simulink model "SimCurtoCircuitoMeioLinhaSemCompensacao"  (R2021b)
settings: Solver=ode45  StartTime=0.0  StopTime=0.1  RelTol=1e-3  EnableMultiTasking=on
values from neighbouring files (symbols this model uses):
  le = 1e-10    [RotinaCurtoCircuitoCompacto.m]    (also in RotinaCurtoCircuitoCompleta.m; RotinaCurtoCircuitoT2F_Trifasico.m)
  lm = (imag(Zm)/(2*pi*f))*d    [RotinaCurtoCircuitoCompacto.m]    (also in RotinaCurtoCircuitoCompleta.m; RotinaCurtoCircuitoT2F_Trifasico.m)
  lp = (imag(Zp)/(2*pi*f))*d    [RotinaCurtoCircuitoCompacto.m]    (also in RotinaCurtoCircuitoCompleta.m; RotinaCurtoCircuitoT2F_Trifasico.m)
  m1 = n    [RotinaCurtoCircuitoCompacto.m]    (also in RotinaCurtoCircuitoCompleta.m; RotinaCurtoCircuitoT2F_Trifasico.m)
  m2 = 1 - m1    [RotinaCurtoCircuitoCompacto.m]    (also in RotinaCurtoCircuitoCompleta.m; RotinaCurtoCircuitoT2F_Trifasico.m)
  NRE = 1e-12    [RotinaCurtoCircuitoCompacto.m]    (also in RotinaCurtoCircuitoCompleta.m; RotinaCurtoCircuitoT2F_Trifasico.m)
  Raf = 1e6    (= 1000000)    [RotinaCurtoCircuitoCompacto.m]    (also in RotinaCurtoCircuitoCompleta.m; RotinaCurtoCircuitoT2F_Trifasico.m = 100000)
  Rbf = 1e6    (= 1000000)    [RotinaCurtoCircuitoCompacto.m]    (also in RotinaCurtoCircuitoCompleta.m; RotinaCurtoCircuitoT2F_Trifasico.m = 1e-05)
  Rcf = 1e6    (= 1000000)    [RotinaCurtoCircuitoCompacto.m]    (also in RotinaCurtoCircuitoCompleta.m; RotinaCurtoCircuitoT2F_Trifasico.m = 1e-05)
  rm = real(Zm)*d    [RotinaCurtoCircuitoCompacto.m]    (also in RotinaCurtoCircuitoCompleta.m; RotinaCurtoCircuitoT2F_Trifasico.m)
  rp = real(Zp)*d    [RotinaCurtoCircuitoCompacto.m]    (also in RotinaCurtoCircuitoCompleta.m; RotinaCurtoCircuitoT2F_Trifasico.m)
  rtc = 10    [RotinaCurtoCircuitoCompacto.m]    (also in RotinaCurtoCircuitoCompleta.m; RotinaCurtoCircuitoT2F_Trifasico.m)
  rti = 10    [RotinaCurtoCircuitoCompacto.m]    (also in RotinaCurtoCircuitoCompleta.m; RotinaCurtoCircuitoT2F_Trifasico.m)
undefined symbols (not defined in the file or in its folder): D11, Delta
libraries: spsSeriesRLCBranchLib x6, spsThreePhaseVIMeasurementLib x2, spsThreePhaseTransformerTwoWindingsLib x2, spsVoltageMeasurementLib x2, spsMutualInductanceLib x2, spsThreePhaseSourceLib x1, spspowerguiLib x1
settings Model: Creator=laris  LastModifiedBy=LeonardoFelipe
settings SolverCC: AlgebraicLoopSolver=TrustRegion
settings DataIOCC: LimitDataPoints=on  SaveFormat=Array  ReturnWorkspaceOutputs=off
settings OptimizationCC: LifeSpan=inf
settings DebuggingCC: SFUnexpectedBacktrackingDiag=warning  SFNoUnconditionalDefaultTransitionDiag=warning  SFExecutionAtInitializationDiag=none  SFMachineParentedDataDiag=warning  ArithmeticOperatorsInVariantConditions=warning
settings HardwareCC: ProdBitPerPointer=32  ProdBitPerSizeT=32  ProdBitPerPtrDiffT=32  ProdLargestAtomicFloat=None  ProdIntDivRoundTo=Undefined  ProdEndianess=Unspecified  ProdWordSize=32  ProdHWDeviceType=32-bit Generic
settings ModelReferenceCC: PropagateSignalLabelsOutOfModel=off
settings SFSimCC: SimUseLocalCustomCode=off  CustomCodeUndefinedFunction=UseInterfaceOnly
settings RTWCC: RTWUseLocalCustomCode=off
settings CodeAppCC: StateflowObjectComments=on
settings GRTTargetCC: TargetLangStandard=C89/C90 (ANSI)
settings ConfigComp: CovMetricSettings=dw  CovSaveCumulativeToWorkspaceVar=on  CovSaveSingleToWorkspaceVar=on  CovExternalEMLEnable=off
settings SimscapeCC: SimscapeNormalizeSystem=off

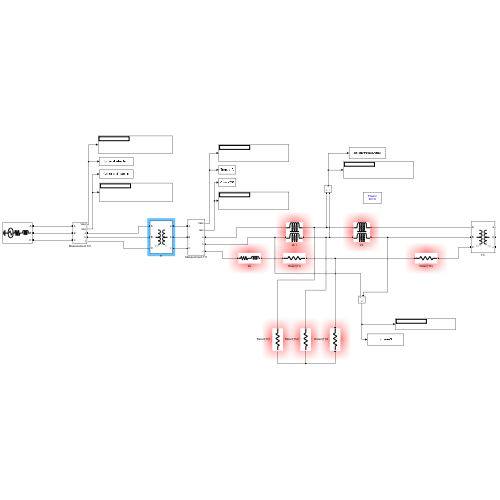
[thumbnail: Simulink's stored preview of the top-level diagram]
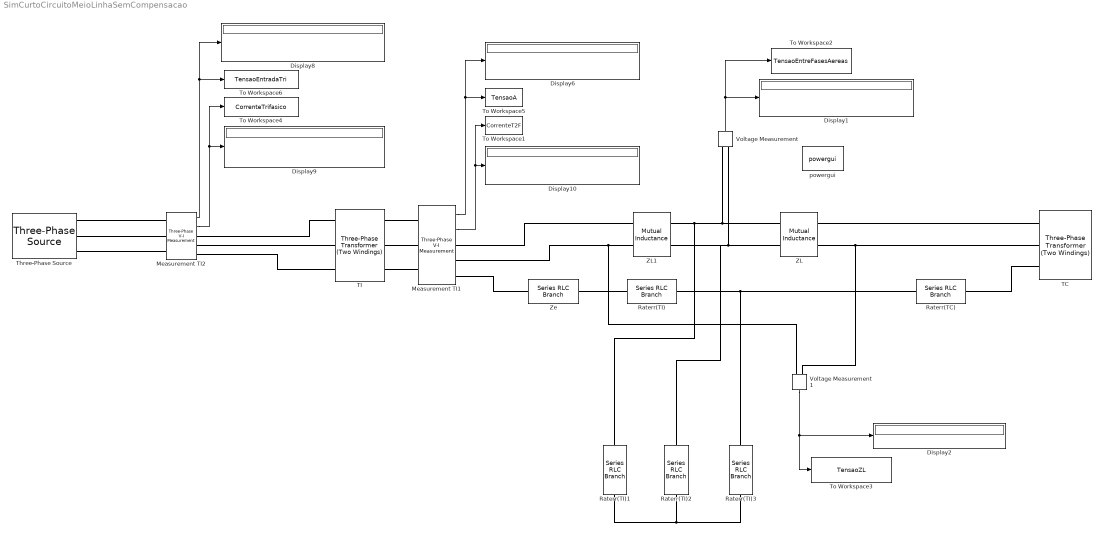
== system SimCurtoCircuitoMeioLinhaSemCompensacao ==
  Display{1..2,6,8..10} (6 alike) : Display
  Measurement TI1 : spsThreePhaseVIMeasurementLib/Three-Phase V-I Measurement  VoltageMeasurement=phase-to-phase  SetLabelV=off  LabelV=Vabc  Vpu=off  VpuLL=off  CurrentMeasurement=yes  SetLabelI=off  LabelI=Iabc  Ipu=off  Pbase=100e6  Vbase=500e3  OutputType=Complex  PhasorSimulation=on  PSBequivalent=0
  Measurement TI2 : spsThreePhaseVIMeasurementLib/Three-Phase V-I Measurement  VoltageMeasurement=phase-to-ground  SetLabelV=off  LabelV=Vabc  Vpu=off  VpuLL=off  CurrentMeasurement=yes  SetLabelI=off  LabelI=Iabc  Ipu=off  Pbase=100e6  Vbase=500e3  OutputType=Complex  PhasorSimulation=on  PSBequivalent=0
  Raterr(TC) : spsSeriesRLCBranchLib/Series RLC Branch  LConnTagsString=__new0  RConnTagsString=__new0  BranchType=R  Resistance=rtc  Inductance=0  SetiL0=off  InitialCurrent=0  Capacitance=1e-6  Setx0=off  InitialVoltage=0  Measurements=None
  Raterr(TI) : spsSeriesRLCBranchLib/Series RLC Branch  LConnTagsString=__new0  RConnTagsString=__new0  BranchType=R  Resistance=rti  Inductance=0  SetiL0=off  InitialCurrent=0  Capacitance=1e-6  Setx0=off  InitialVoltage=0  Measurements=None
  Raterr(TI)1 : spsSeriesRLCBranchLib/Series RLC Branch  LConnTagsString=__new0  RConnTagsString=__new0  BranchType=R  Resistance=Raf  Inductance=0  SetiL0=off  InitialCurrent=0  Capacitance=1e-6  Setx0=off  InitialVoltage=0  Measurements=None
  Raterr(TI)2 : spsSeriesRLCBranchLib/Series RLC Branch  LConnTagsString=__new0  RConnTagsString=__new0  BranchType=R  Resistance=Rbf  Inductance=0  SetiL0=off  InitialCurrent=0  Capacitance=1e-6  Setx0=off  InitialVoltage=0  Measurements=None
  Raterr(TI)3 : spsSeriesRLCBranchLib/Series RLC Branch  LConnTagsString=__new0  RConnTagsString=__new0  BranchType=R  Resistance=Rcf  Inductance=0  SetiL0=off  InitialCurrent=0  Capacitance=1e-6  Setx0=off  InitialVoltage=0  Measurements=None
  TC : spsThreePhaseTransformerTwoWindingsLib/Three-Phase Transformer (Two Windings)  Winding1Connection=Delta (D11)  Winding2Connection=Yg  CoreType=Three single-phase transformers  SetSaturation=off  Hysteresis=off  DataFile='hysteresis'  SetInitialFlux=off  Measurements=None  UNITS=pu  NominalPower=[120e3 , 60]  Winding1=[13800 0.0048118 0.018511]  Winding2=[380 0.0048119 0.018511]  Rm=5.801193266567229e+02*1000  Lm=8.409977380031759e+02*1000  L0=0.50001  Saturation=[0 0;0.0012545 0.01913;0.52272 0.024231]  InitialFluxes=[0.66025 -0.66025 0.57767]  BreakLoop=off  DiscreteSolver=Trapezoidal iterative  DataType=off  TransfoNumber=1
  TI : spsThreePhaseTransformerTwoWindingsLib/Three-Phase Transformer (Two Windings)  Winding1Connection=Delta (D11)  Winding2Connection=Y  CoreType=Three single-phase transformers  SetSaturation=off  Hysteresis=off  DataFile='hysteresis'  SetInitialFlux=off  Measurements=None  UNITS=pu  NominalPower=[300e3 , 60 ]  Winding1=[13800 0.0048119 0.018511]  Winding2=[13800 0.0048119 0.018511]  Rm=1.730769230769231e+03*1000  Lm=40.010686750359440*1000  L0=6.3145  Saturation=[0 0;0.0012545 0.01913;0.52272 0.024231]  InitialFluxes=[34.179 -34.179 29.906]  BreakLoop=off  DiscreteSolver=Trapezoidal iterative  DataType=off  TransfoNumber=1
  Three-Phase Source : spsThreePhaseSourceLib/Three-Phase Source  InternalConnection=Yg  VoltagePhases=off  Voltage=13.8e3  PhaseAngle=0  Voltage_phases=[25e3 25e3 25e3]/sqrt(3)  PhaseAngles_phases=[0 -120 +120]  Frequency=60  NonIdealSource=on  SpecifyImpedance=on  Resistance=0.8929  Inductance=16.58e-3  ShortCircuitLevel=120e6  BaseVoltage=13.8e3  XRratio=7  BusType=swing  Pref=10e3  Qref=0  Prefabc=[10e3, 10e3, 10e3]  Qrefabc=[0, 0, 0]  Qmin=-inf  Qmax=inf
  To Workspace1 : ToWorkspace  VariableName=CorrenteT2F  SampleTime=-1
      settings: MaxDataPoints=1
  To Workspace2 : ToWorkspace  VariableName=TensaoEntreFasesAereas  SampleTime=-1
      settings: MaxDataPoints=1
  To Workspace3 : ToWorkspace  VariableName=TensaoZL  SampleTime=-1
      settings: MaxDataPoints=1
  To Workspace4 : ToWorkspace  VariableName=CorrenteTrifasico  SampleTime=-1
      settings: MaxDataPoints=1
  To Workspace5 : ToWorkspace  VariableName=TensaoA  SampleTime=-1
      settings: MaxDataPoints=1
  To Workspace6 : ToWorkspace  VariableName=TensaoEntradaTri  SampleTime=-1
      settings: MaxDataPoints=1
  Voltage Measurement : spsVoltageMeasurementLib/Voltage Measurement  PhasorSimulation=on  OutputType=Complex  PSBequivalent=0
  Voltage Measurement1 : spsVoltageMeasurementLib/Voltage Measurement  PhasorSimulation=on  OutputType=Complex  PSBequivalent=0
  ZL : spsMutualInductanceLib/Mutual Inductance  LConnTagsString=a|b  RConnTagsString=A|B  TypeOfMutual=Generalized mutual inductance  NumberOfWindings=2  SelfImpedance1=[1.1 1.1e-03]  SelfImpedance2=[ 1.1 1.1e-03]  ThreeWindings=on  SelfImpedance3=[ 1.1 1.1e-03]  MutualImpedance=[1.0 1.0e-03]  InductanceMatrix=[lp lm ; lm lp] * m2  ResistanceMatrix=[rp rm ; rm rp] * m2  Measurements=None
      settings: SourceProductBaseCode=PS
  ZL1 : spsMutualInductanceLib/Mutual Inductance  LConnTagsString=a|b  RConnTagsString=A|B  TypeOfMutual=Generalized mutual inductance  NumberOfWindings=2  SelfImpedance1=[1.1 1.1e-03]  SelfImpedance2=[ 1.1 1.1e-03]  ThreeWindings=on  SelfImpedance3=[ 1.1 1.1e-03]  MutualImpedance=[1.0 1.0e-03]  InductanceMatrix=[lp lm ; lm lp] * m1  ResistanceMatrix=[rp rm ; rm rp] * m1  Measurements=None
      settings: SourceProductBaseCode=PS
  Ze : spsSeriesRLCBranchLib/Series RLC Branch  LConnTagsString=__new0  RConnTagsString=__new0  BranchType=RL  Resistance=NRE  Inductance=le  SetiL0=off  InitialCurrent=0  Capacitance=le  Setx0=off  InitialVoltage=0  Measurements=None
  powergui : spspowerguiLib/powergui  Priority=1  SimulationMode=Phasor  SampleTime=50e-6  frequency=60  Iterations=50  frequencyindice=60  Pbase=100e6  ErrMax=1e-4  UnitsV=kV  UnitsW=MW  buscounter=0  FunctionMessages=off  echomessages=off  EnableUseOfTLC=off  CurrentSourceSwitches=off  DisableSnubberDevices=off  DisableRonSwitches=off  DisableVfSwitches=off  DisplayEquations=off  AutomaticDiscreteSolvers=off  SolverType=Tustin/Backward Euler (TBE)  Interpol=off  ExternalGateDelay=off  methode=off  Ts=100  x0status=blocks  SPID=on  SwTol=0  HookPort=off  NonlinearTolerance=1e-4  nMaxIteration=100  ContinueOnMaxIteration=off  RestoreLinks=warning  ResistiveCurrentMeasurement=off  Frange=[0:2:500]  Ylog=off  Xlog=on  ShowGrid=off  save=off  variable=ZData  structure=0  ZoomFFT=off  StartTime=0.0  cycles=1  DisplayStyle=1  fundamental=60  FreqAxis=off  MaxFrequency=1000  frequencyindicesteady=1  RmsSteady=1  display=off
  wires:
  Measurement TI1/1 -> To Workspace5/1, Display6/1
  Measurement TI2/1 -> Display8/1, To Workspace6/1
  Measurement TI2/2 -> To Workspace4/1, Display9/1
  Measurement TI1/2 -> To Workspace1/1, Display10/1
  Voltage Measurement/1 -> To Workspace2/1, Display1/1
  Voltage Measurement1/1 -> To Workspace3/1, Display2/1
  connections:
  ZL/RConn1 -- TC/LConn1
  ZL/RConn2 -- Voltage Measurement1/LConn2 -- TC/LConn2
  Raterr(TC)/RConn1 -- TC/LConn3
  TI/RConn1 -- Measurement TI1/LConn1
  Voltage Measurement/LConn1 -- ZL1/RConn1 -- Raterr(TI)1/LConn1 -- ZL/LConn1
  Voltage Measurement/LConn2 -- ZL/LConn2 -- Raterr(TI)2/LConn1 -- ZL1/RConn2
  Ze/LConn1 -- Measurement TI1/RConn3
  Three-Phase Source/RConn3 -- Measurement TI2/LConn3
  Three-Phase Source/RConn2 -- Measurement TI2/LConn2
  Three-Phase Source/RConn1 -- Measurement TI2/LConn1
  Raterr(TI)1/RConn1 -- Raterr(TI)3/RConn1 -- Raterr(TI)2/RConn1
  TI/LConn1 -- Measurement TI2/RConn1
  TI/LConn2 -- Measurement TI2/RConn2
  TI/LConn3 -- Measurement TI2/RConn3
  Measurement TI1/LConn2 -- TI/RConn2
  Measurement TI1/LConn3 -- TI/RConn3
  Ze/RConn1 -- Raterr(TI)/LConn1
  Raterr(TI)/RConn1 -- Raterr(TI)3/LConn1 -- Raterr(TC)/LConn1
  Measurement TI1/RConn1 -- ZL1/LConn1
  ZL1/LConn2 -- Voltage Measurement1/LConn1 -- Measurement TI1/RConn2
